simulink model "ASLIPtail"  (R2015a)
settings: Solver=ode45  StartTime=0.0  StopTime=500  MaxStep=1e-3  RelTol=1e-4  AbsTol=1e-6
values from neighbouring files (symbols this model uses):
  a0 = 67*pi/180    (= 1.16937059884)    [ASLIPrun_params2.m]
  dt0 = deg2rad(0)    [ASLIPrun_params2.m]
  dx0 = 5.00    (= 5)    [ASLIPrun_params2.m]
  dy0 = 0    [ASLIPrun_params2.m]
  g = 9.81    [ASLIPrun_params2.m]
  J = 4.58    [ASLIPrun_params2.m]
  k = 20000    [ASLIPrun_params2.m]
  kt = 100    [ASLIPrun_params2.m]
  L = 0.1    [ASLIPrun_params2.m]    (also in AnimSMR2.m = sqrt( (u(4)-u(9))^2 + (u(5)-u(10))^2 ))
  l0 = 1    [ASLIPrun_params2.m]
  m = 80    [ASLIPrun_params2.m]
  model = 1    [ASLIPrun_params2.m]
  r0 = sqrt(xr0^2 + yr0^2)    [ASLIPrun_params2.m]
  rp = 0.005    [ASLIPrun_params2.m]
  t0 = 70*pi/180    (= 1.2217304764)    [ASLIPrun_params2.m]
  x0 = 0*(-l0 + L*cos(t0))    [ASLIPrun_params2.m]    (also in AnimSMR2.m = [])
  xr0 = -l0*cos(a0) + L*cos(t0)    [ASLIPrun_params2.m]
  y0 = 1.065    [ASLIPrun_params2.m]
  yr0 = l0*sin(a0) + L*sin(t0)    [ASLIPrun_params2.m]
libraries: simulink_extras x1
settings Model: Creator=hgeyer  LastModifiedBy=Joe
settings DataIOCC: LimitDataPoints=off  SignalLoggingSaveFormat=ModelDataLogs
settings OptimizationCC: ExpressionDepthLimit=2147483647
settings DebuggingCC: UnderspecifiedInitializationDetection=Classic  MergeDetectMultiDrivingBlocksExec=none  SolverPrmCheckMsg=warning  FcnCallInpInsideContextMsg=EnableAllAsWarning  StateNameClashWarn=warning

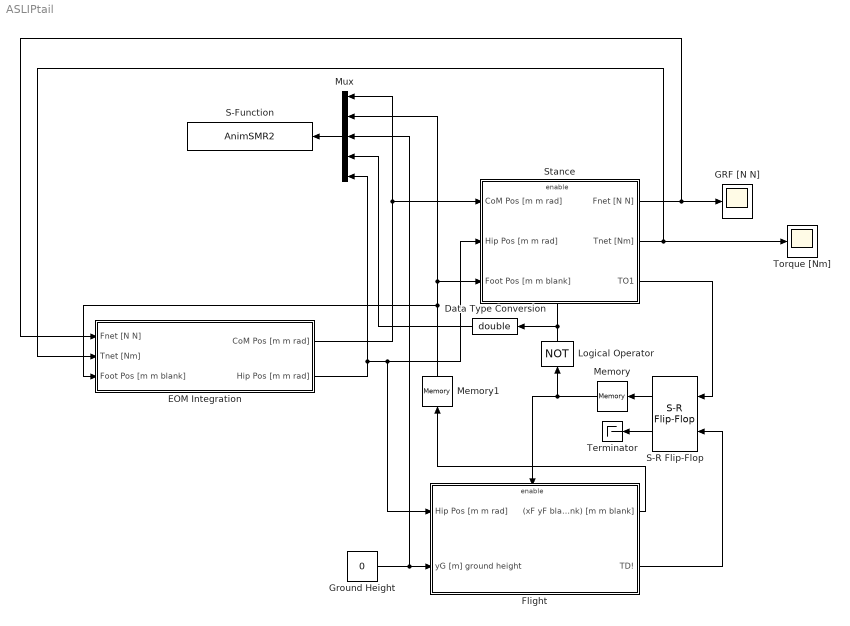
== system ASLIPtail ==
  Data Type Conversion : DataTypeConversion  OutDataTypeStr=double
  EOM Integration : Subsystem
  Flight : Subsystem
  GRF [N N] : Scope
      settings: TimeRange=8  YMin=-500  YMax=2250  MaxDataPoints=50000
  Ground Height : Constant  Value=0
  Logical Operator : Logic  Operator=NOT  AllPortsSameDT=off  OutDataTypeStr=boolean
  Memory : Memory  X0=1
  Memory1 : Memory  X0="[(x0 - xr0) (y0 - yr0)  0]"
  Mux : Mux  Inputs=5
  S-Function : S-Function  FunctionName=AnimSMR2  Parameters=0.005
  S-R Flip-Flop : simulink_extras/Flip Flops/S-R Flip-Flop  initial_condition=1
  Stance : Subsystem
  Terminator : Terminator
  Torque [Nm] : Scope
      settings: YMin=-10  YMax=10  SaveName=ScopeData3
  wires:
  EOM Integration/1(CoM Pos [m m rad]) -> Stance/1("CoM Pos [m m rad] "), Mux/1
  Stance/3(TO1) -> S-R Flip-Flop/1
  S-R Flip-Flop/1 -> Memory/1
  Logical Operator/1 -> Data Type Conversion/1, Stance/Enable
  Memory/1 -> Logical Operator/1, Flight/Enable
  Flight/2(TD!) -> S-R Flip-Flop/2
  Stance/1(Fnet [N N]) -> EOM Integration/1(Fnet [N N]), GRF [N N]/1
  Flight/1((xF yF blank) [m m blank]) -> Memory1/1
  Memory1/1 -> EOM Integration/3(Foot Pos [m m blank]), Mux/2, Stance/3(Foot Pos [m m blank])
  Mux/1 -> S-Function/1
  S-R Flip-Flop/2 -> Terminator/1
  Ground Height/1 -> Mux/3, Flight/2(yG [m] ground height)
  Data Type Conversion/1 -> Mux/4
  EOM Integration/2(Hip Pos [m m rad]) -> Mux/5, Stance/2(Hip Pos [m m rad]), Flight/1(Hip Pos [m m rad])
  Stance/2(Tnet [Nm]) -> Torque [Nm]/1, EOM Integration/2(Tnet [Nm])

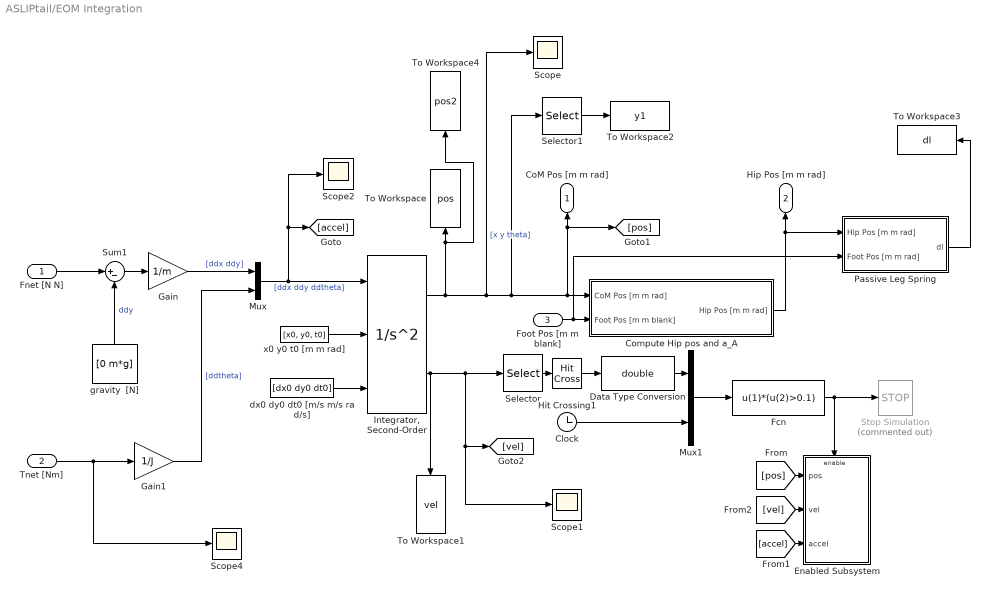
== system ASLIPtail/EOM Integration ==
  Fnet [N N] : Inport
  Tnet [Nm] : Inport  Port=2
  Foot Pos [m m blank] : Inport  Port=3
  Clock : Clock
  Compute Hip pos and a_A : Subsystem
  Data Type Conversion : DataTypeConversion  OutDataTypeStr=double
  Enabled Subsystem : Subsystem  TreatAsAtomicUnit=on
  Fcn : Fcn  Expr=u(1)*(u(2)>0.1)
  Gain : Gain  Gain=1/m
  Gain1 : Gain  Gain=1/J
  Hit Crossing1 : HitCross  HitCrossingDirection=falling
  "Integrator, Second-Order" : SecondOrderIntegrator  ICSourceX=external  ICSourceDXDT=external
  Mux : Mux  Inputs=2
  Mux1 : Mux  Inputs=2
  Passive Leg Spring : Subsystem
  Scope{,1..2,4} (4 alike) : Scope
      Scope settings: TimeRange=50  YMin=-0  YMax=250  SaveName=ScopeData7  MaxDataPoints=500000
      Scope1 settings: YMin=-1  YMax=5.5  SaveName=ScopeData8  MaxDataPoints=500000
      Scope2 settings: TimeRange=50  YMin=-0  YMax=250  SaveName=ScopeData13  MaxDataPoints=500000
      Scope4 settings: YMin=-1  YMax=5.5  SaveName=ScopeData16  MaxDataPoints=500000
  Selector : Selector  InputPortWidth=3  Indices=[2]
  Selector1 : Selector  InputPortWidth=3  Indices=[2]
  Stop Simulation : Stop  Commented=on
  Sum1 : Sum  Inputs=|+-
  To Workspace : ToWorkspace  VariableName=pos  SampleTime=-1
  To Workspace1 : ToWorkspace  VariableName=vel  SampleTime=-1
  To Workspace2 : ToWorkspace  VariableName=y1  SaveFormat=Structure With Time  SampleTime=-1
  To Workspace3 : ToWorkspace  VariableName=dl  SampleTime=-1
  To Workspace4 : ToWorkspace  VariableName=pos2  SaveFormat=Timeseries  SampleTime=-1
  dx0 dy0 dt0 [m/s m/s ra d/s] : Constant  Value=[dx0 dy0 dt0]
  gravity  [N] : Constant  Value=[0 m*g]
  x0 y0 t0 [m m rad] : Constant  Value=[x0, y0, t0]
  CoM Pos [m m rad] : Outport
  Hip Pos [m m rad] : Outport  Port=2
  wires:
  Sum1/1 -> Gain/1
  gravity  [N]/1 -> Sum1/2  "ddy"
  x0 y0 t0 [m m rad]/1 -> "Integrator, Second-Order"/2
  Gain/1 -> Mux/1  "[ddx ddy]"
  Fnet [N N]/1 -> Sum1/1
  dx0 dy0 dt0 [m/s m/s ra d/s]/1 -> "Integrator, Second-Order"/3
  Mux/1 -> [accel], Scope2/1, "Integrator, Second-Order"/1  "[ddx ddy ddtheta]"
  Gain1/1 -> Mux/2  "[ddtheta]"
  Tnet [Nm]/1 -> Scope4/1, Gain1/1
  "Integrator, Second-Order"/1 -> Scope/1, Selector1/1, Compute Hip pos and a_A/1(CoM Pos [m m rad]), [pos], CoM Pos [m m rad]/1, To Workspace4/1, To Workspace/1  "[x y theta]"
  Foot Pos [m m blank]/1 -> Passive Leg Spring/2(Foot Pos [m m rad]), Compute Hip pos and a_A/2(Foot Pos [m m blank])
  Compute Hip pos and a_A/1(Hip Pos [m m rad]) -> Hip Pos [m m rad]/1, Passive Leg Spring/1(Hip Pos [m m rad])
  Hit Crossing1/1 -> Data Type Conversion/1
  Clock/1 -> Mux1/2
  Mux1/1 -> Fcn/1
  Fcn/1 -> Stop Simulation/1, Enabled Subsystem/Enable
  Data Type Conversion/1 -> Mux1/1
  "Integrator, Second-Order"/2 -> Scope1/1, [vel], Selector/1, To Workspace1/1
  Selector/1 -> Hit Crossing1/1
  Selector1/1 -> To Workspace2/1
  Passive Leg Spring/1(dl) -> To Workspace3/1
  [accel] -> Enabled Subsystem/3(accel)
  [pos] -> Enabled Subsystem/1(pos)
  [vel] -> Enabled Subsystem/2(vel)

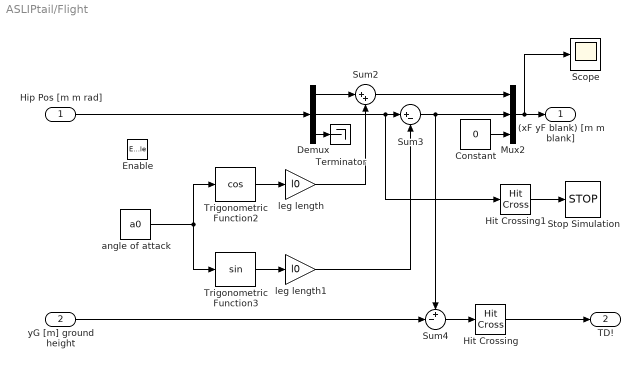
== system ASLIPtail/Flight ==
  Hip Pos [m m rad] : Inport
  yG [m] ground height : Inport  Port=2
  Enable : EnablePort  StatesWhenEnabling=reset
  Constant : Constant  Value=0
  Demux : Demux  Outputs=3
  Hit Crossing : HitCross  HitCrossingDirection=falling
  Hit Crossing1 : HitCross  HitCrossingDirection=falling
  Mux2 : Mux  Inputs=3
  Scope : Scope
      settings: SaveName=ScopeData11
  Stop Simulation : Stop
  Sum2 : Sum  Inputs=|++
  Sum3 : Sum  Inputs=|+-
  Sum4 : Sum  Inputs=+-|
  Terminator : Terminator
  Trigonometric Function2 : Trigonometry  Operator=cos
  Trigonometric Function3 : Trigonometry
  angle of attack : Constant  Value=a0
  leg length : Gain  Gain=l0
  leg length1 : Gain  Gain=l0
  (xF yF blank) [m m blank] : Outport  InitialOutput=[0 0 0]
      settings: AttributesFormatString=%<OutputWhenDisabled>
  TD! : Outport  Port=2  OutputWhenDisabled=reset  InitialOutput=0
      settings: AttributesFormatString=%<OutputWhenDisabled>
  wires:
  Hit Crossing/1 -> TD!/1
  Demux/2 -> Hit Crossing1/1, Sum3/1
  Demux/1 -> Sum2/1
  angle of attack/1 -> Trigonometric Function3/1, Trigonometric Function2/1
  Trigonometric Function2/1 -> leg length/1
  Trigonometric Function3/1 -> leg length1/1
  Hip Pos [m m rad]/1 -> Demux/1
  leg length/1 -> Sum2/2
  leg length1/1 -> Sum3/2
  Sum3/1 -> Mux2/2, Sum4/1
  Sum2/1 -> Mux2/1
  Mux2/1 -> Scope/1, (xF yF blank) [m m blank]/1
  yG [m] ground height/1 -> Sum4/2
  Sum4/1 -> Hit Crossing/1
  Constant/1 -> Mux2/3
  Hit Crossing1/1 -> Stop Simulation/1
  Demux/3 -> Terminator/1

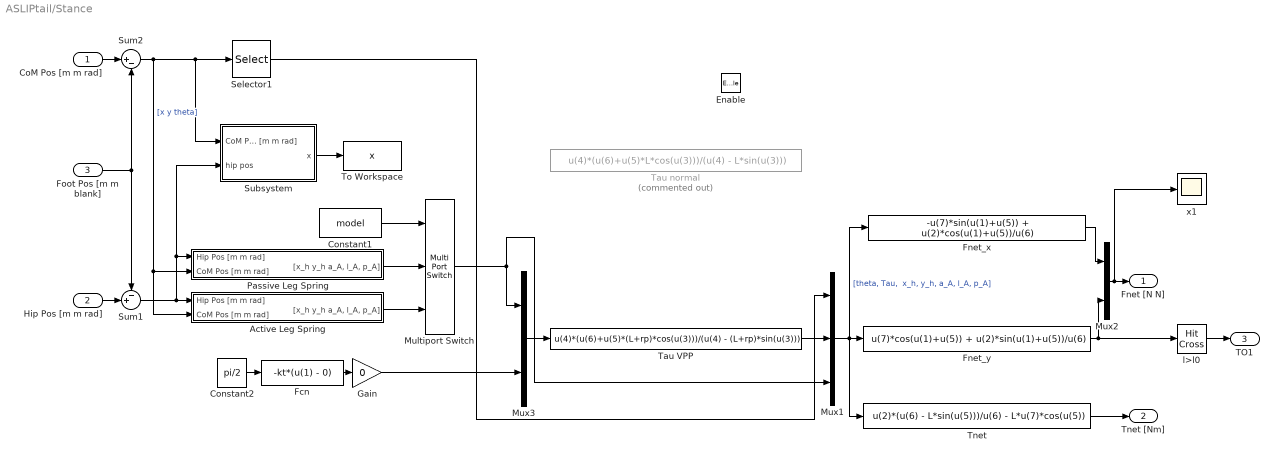
== system ASLIPtail/Stance ==
  "CoM Pos [m m rad] " : Inport
  Hip Pos [m m rad] : Inport  Port=2
  Foot Pos [m m blank] : Inport  Port=3
  Enable : EnablePort  StatesWhenEnabling=reset
  Active Leg Spring : Subsystem
  Constant1 : Constant  Value=model
  Constant2 : Constant  Value=pi/2
  Fcn : Fcn  Expr=-kt*(u(1) - 0)
  Fnet_x : Fcn  Expr=-u(7)*sin(u(1)+u(5)) + u(2)*cos(u(1)+u(5))/u(6)
  Fnet_y : Fcn  Expr=u(7)*cos(u(1)+u(5)) + u(2)*sin(u(1)+u(5))/u(6)
  Gain : Gain  Gain=0
  Multiport Switch : MultiPortSwitch  Inputs=2
  Mux1 : Mux  Inputs=3
  Mux2 : Mux  Inputs=2
  Mux3 : Mux  Inputs=2
  Passive Leg Spring : Subsystem
  Selector1 : Selector  InputPortWidth=3  Indices=[3]
  Subsystem : Subsystem
  Sum1 : Sum  Inputs=-+|
  Sum2 : Sum  Inputs=|+-
  Tau VPP : Fcn  Expr=u(4)*(u(6)+u(5)*(L+rp)*cos(u(3)))/(u(4) - (L+rp)*sin(u(3)))
  Tau normal : Fcn  Commented=on  Expr=u(4)*(u(6)+u(5)*L*cos(u(3)))/(u(4) - L*sin(u(3)))
  Tnet : Fcn  Expr=u(2)*(u(6) - L*sin(u(5)))/u(6) - L*u(7)*cos(u(5))
  To Workspace : ToWorkspace  VariableName=x  SampleTime=-1
  l>l0 : HitCross  HitCrossingOffset=l0  HitCrossingDirection=falling
  x1 : Scope
      settings: YMin=-9  YMax=8  SaveName=ScopeData12  MaxDataPoints=500
  Fnet [N N] : Outport  OutputWhenDisabled=reset  InitialOutput=[0,0]
  Tnet [Nm] : Outport  Port=2  OutputWhenDisabled=reset  InitialOutput=[0]
  TO1 : Outport  Port=3  OutputWhenDisabled=reset  InitialOutput=[0]
  wires:
  Tau VPP/1 -> Mux1/2
  Selector1/1 -> Mux1/1
  Fnet_x/1 -> Mux2/1
  Tnet/1 -> Tnet [Nm]/1
  "CoM Pos [m m rad] "/1 -> Sum2/1
  Sum1/1 -> Subsystem/2(hip pos), Passive Leg Spring/1(Hip Pos [m m rad]), Active Leg Spring/1(Hip Pos [m m rad])
  Hip Pos [m m rad]/1 -> Sum1/2
  Mux1/1 -> Tnet/1, Fnet_x/1, Fnet_y/1  "[theta, Tau,  x_h, y_h, a_A, l_A, p_A]"
  Foot Pos [m m blank]/1 -> Sum1/1, Sum2/2
  Sum2/1 -> Active Leg Spring/2(CoM Pos [m m rad]), Passive Leg Spring/2(CoM Pos [m m rad]), Subsystem/1(CoM Pos [m m rad]), Selector1/1  "[x y theta]"
  Mux2/1 -> x1/1, Fnet [N N]/1
  Fnet_y/1 -> l>l0/1, Mux2/2
  l>l0/1 -> TO1/1
  Mux3/1 -> Tau VPP/1
  Multiport Switch/1 -> Mux3/1, Mux1/3
  Gain/1 -> Mux3/2
  Fcn/1 -> Gain/1
  Passive Leg Spring/1("[x_h y_h a_A, l_A, p_A]") -> Multiport Switch/2
  Active Leg Spring/1("[x_h y_h a_A, l_A, p_A]") -> Multiport Switch/3
  Constant1/1 -> Multiport Switch/1
  Constant2/1 -> Fcn/1
  Subsystem/1(x) -> To Workspace/1

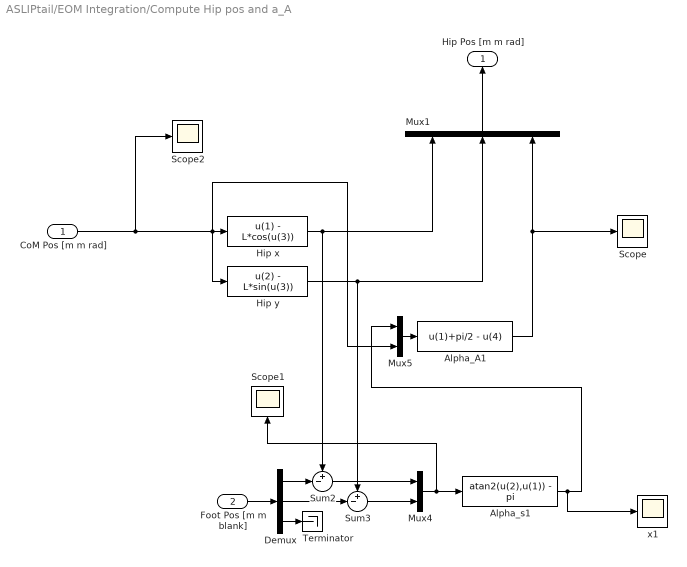
== system ASLIPtail/EOM Integration/Compute Hip pos and a_A ==
  CoM Pos [m m rad] : Inport
  Foot Pos [m m blank] : Inport  Port=2
  Alpha_A1 : Fcn  Expr=u(1)+pi/2 - u(4)
  Alpha_s1 : Fcn  Expr=atan2(u(2),u(1)) - pi
  Demux : Demux  Outputs=3
  Hip x : Fcn  Expr=u(1) - L*cos(u(3))
  Hip y : Fcn  Expr=u(2) - L*sin(u(3))
  Mux1 : Mux  Inputs=3
  Mux4 : Mux  Inputs=2
  Mux5 : Mux  Inputs=2
  Scope : Scope
      settings: TimeRange=5  SaveName=ScopeData2
  Scope1 : Scope
  Scope2 : Scope
      settings: SaveName=ScopeData9
  Sum2 : Sum  Inputs=+-|
  Sum3 : Sum  Inputs=+-|
  Terminator : Terminator
  x1 : Scope
      settings: SaveName=ScopeData4
  Hip Pos [m m rad] : Outport
  wires:
  CoM Pos [m m rad]/1 -> Scope2/1, Hip x/1, Hip y/1, Mux5/2
  Mux4/1 -> Alpha_s1/1, Scope1/1
  Mux5/1 -> Alpha_A1/1
  Hip x/1 -> Sum2/1, Mux1/1
  Mux1/1 -> Hip Pos [m m rad]/1
  Hip y/1 -> Sum3/1, Mux1/2
  Alpha_s1/1 -> x1/1, Mux5/1
  Demux/2 -> Sum3/2
  Demux/3 -> Terminator/1
  Sum2/1 -> Mux4/1
  Demux/1 -> Sum2/2
  Alpha_A1/1 -> Mux1/3, Scope/1
  Foot Pos [m m blank]/1 -> Demux/1
  Sum3/1 -> Mux4/2

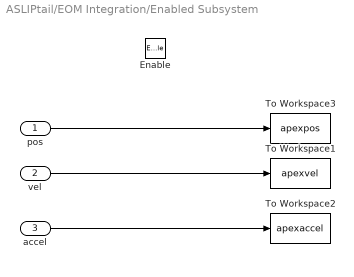
== system ASLIPtail/EOM Integration/Enabled Subsystem ==
  pos : Inport
  vel : Inport  Port=2
  accel : Inport  Port=3
  Enable : EnablePort
  To Workspace1 : ToWorkspace  VariableName=apexvel  SaveFormat=Timeseries  SampleTime=-1
  To Workspace2 : ToWorkspace  VariableName=apexaccel  SaveFormat=Timeseries  SampleTime=-1
  To Workspace3 : ToWorkspace  VariableName=apexpos  SaveFormat=Timeseries  SampleTime=-1
  wires:
  pos/1 -> To Workspace3/1
  vel/1 -> To Workspace1/1
  accel/1 -> To Workspace2/1

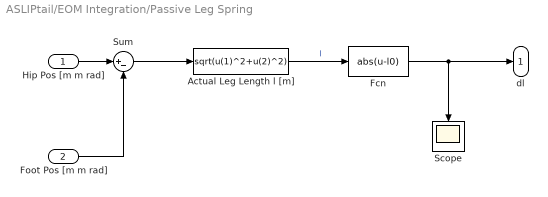
== system ASLIPtail/EOM Integration/Passive Leg Spring ==
  Hip Pos [m m rad] : Inport
  Foot Pos [m m rad] : Inport  Port=2
  Actual Leg Length l [m] : Fcn  Expr=sqrt(u(1)^2+u(2)^2)
  Fcn : Fcn  Expr=abs(u-l0)
  Scope : Scope
      settings: SaveName=ScopeData14
  Sum : Sum  Inputs=|+-
  dl : Outport
  wires:
  Actual Leg Length l [m]/1 -> Fcn/1  "l"
  Foot Pos [m m rad]/1 -> Sum/2
  Fcn/1 -> dl/1, Scope/1
  Hip Pos [m m rad]/1 -> Sum/1
  Sum/1 -> Actual Leg Length l [m]/1

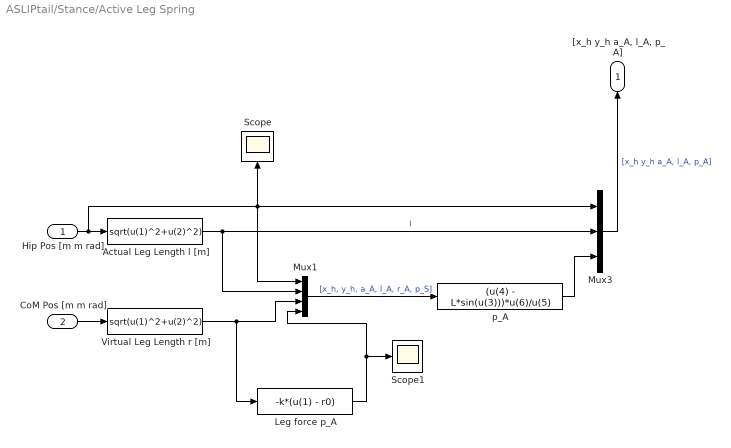
== system ASLIPtail/Stance/Active Leg Spring ==
  Hip Pos [m m rad] : Inport
  CoM Pos [m m rad] : Inport  Port=2
  Actual Leg Length l [m] : Fcn  Expr=sqrt(u(1)^2+u(2)^2)
  Leg force p_A : Fcn  Expr=-k*(u(1) - r0)
  Mux1 : Mux
  Mux3 : Mux  Inputs=3
  Scope : Scope
      settings: SaveName=ScopeData2
  Scope1 : Scope
      settings: SaveName=ScopeData5
  Virtual Leg Length r [m] : Fcn  Expr=sqrt(u(1)^2+u(2)^2)
  p_A : Fcn  Expr=(u(4) - L*sin(u(3)))*u(6)/u(5)
  "[x_h y_h a_A, l_A, p_A]" : Outport
  wires:
  CoM Pos [m m rad]/1 -> Virtual Leg Length r [m]/1
  p_A/1 -> Mux3/3
  Mux1/1 -> p_A/1  "[x_h, y_h, a_A, l_A, r_A, p_S]"
  Virtual Leg Length r [m]/1 -> Mux1/3, Leg force p_A/1
  Hip Pos [m m rad]/1 -> Mux1/1, Mux3/1, Scope/1, Actual Leg Length l [m]/1
  Actual Leg Length l [m]/1 -> Mux3/2, Mux1/2  "l"
  Mux3/1 -> "[x_h y_h a_A, l_A, p_A]"/1  "[x_h y_h a_A, l_A, p_A]"
  Leg force p_A/1 -> Scope1/1, Mux1/4

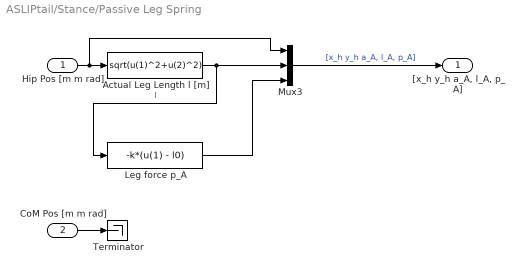
== system ASLIPtail/Stance/Passive Leg Spring ==
  Hip Pos [m m rad] : Inport
  CoM Pos [m m rad] : Inport  Port=2
  Actual Leg Length l [m] : Fcn  Expr=sqrt(u(1)^2+u(2)^2)
  Leg force p_A : Fcn  Expr=-k*(u(1) - l0)
  Mux3 : Mux  Inputs=3
  Terminator : Terminator
  "[x_h y_h a_A, l_A, p_A]" : Outport
  wires:
  Mux3/1 -> "[x_h y_h a_A, l_A, p_A]"/1  "[x_h y_h a_A, l_A, p_A]"
  Actual Leg Length l [m]/1 -> Leg force p_A/1, Mux3/2  "l"
  Leg force p_A/1 -> Mux3/3
  Hip Pos [m m rad]/1 -> Actual Leg Length l [m]/1, Mux3/1
  CoM Pos [m m rad]/1 -> Terminator/1

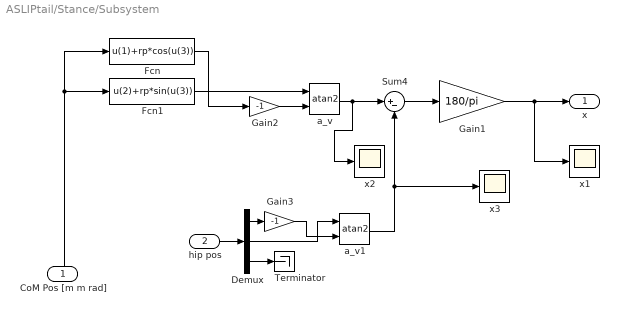
== system ASLIPtail/Stance/Subsystem ==
  CoM Pos [m m rad] : Inport
  hip pos : Inport  Port=2
  Demux : Demux  Outputs=3
  Fcn : Fcn  Expr=u(1)+rp*cos(u(3))
  Fcn1 : Fcn  Expr=u(2)+rp*sin(u(3))
  Gain1 : Gain  Gain=180/pi
  Gain2 : Gain  Gain=-1
  Gain3 : Gain  Gain=-1
  Sum4 : Sum  Inputs=|+-
  Terminator : Terminator
  a_v : Trigonometry  Operator=atan2
  a_v1 : Trigonometry  Operator=atan2
  x1 : Scope
      settings: YMin=-3.5  YMax=3.5  SaveName=ScopeData6  MaxDataPoints=500
  x2 : Scope
      settings: YMin=-3.5  YMax=3.5  SaveName=ScopeData10  MaxDataPoints=500
  x3 : Scope
      settings: YMin=-3.5  YMax=3.5  SaveName=ScopeData17  MaxDataPoints=500
  x : Outport
  wires:
  Sum4/1 -> Gain1/1
  a_v/1 -> x2/1, Sum4/1
  Fcn/1 -> Gain2/1
  Gain2/1 -> a_v/2
  Fcn1/1 -> a_v/1
  Gain1/1 -> x1/1, x/1
  CoM Pos [m m rad]/1 -> Fcn1/1, Fcn/1
  hip pos/1 -> Demux/1
  Demux/1 -> Gain3/1
  Demux/2 -> a_v1/1
  Gain3/1 -> a_v1/2
  a_v1/1 -> x3/1, Sum4/2
  Demux/3 -> Terminator/1
